simulink model "hw2Q7_model"  (R2021a)
settings: Solver=VariableStepAuto  StartTime=0.0  StopTime=time_end  RelTol=1e-3
values from neighbouring files (symbols this model uses):
  alpha = 60    [hw2Q7.m]
  E = 720    [hw2Q7.m]
  F = 180    [hw2Q7.m]
  K1 = (1 + G * K2) / G    [hw2Q7.m]
  K2 = K2_list{i}    [hw2Q7.m]
  m = 1000    [hw2Q7.m]
settings Model: Creator=kaiyu  LastModifiedBy=kaiyu

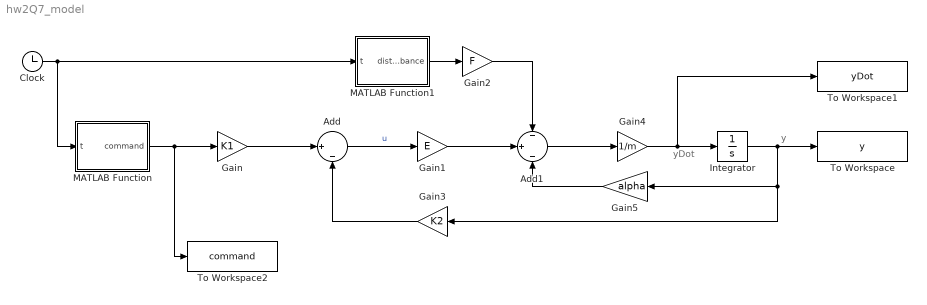
== system hw2Q7_model ==
  note: yDot
  note: y
  Add : Sum  Inputs=||+|-
  Add1 : Sum  Inputs=-|+|-
  Clock : Clock
  Gain : Gain  Gain=K1
  Gain1 : Gain  Gain=E
  Gain2 : Gain  Gain=F
  Gain3 : Gain  Gain=K2
  Gain4 : Gain  Gain=1/m
  Gain5 : Gain  Gain=alpha
  Integrator : Integrator  InitialCondition=20
  MATLAB Function : MATLAB Function  TreatAsAtomicUnit=on
  MATLAB Function1 : MATLAB Function  TreatAsAtomicUnit=on
  To Workspace : ToWorkspace  VariableName=y  SaveFormat=Timeseries  SampleTime=-1
  To Workspace1 : ToWorkspace  VariableName=yDot  SaveFormat=Timeseries  SampleTime=-1
  To Workspace2 : ToWorkspace  VariableName=command  SaveFormat=Timeseries  SampleTime=-1
  wires:
  Gain/1 -> Add/1
  Add/1 -> Gain1/1  "u"
  Gain1/1 -> Add1/2
  Gain2/1 -> Add1/1
  MATLAB Function1/1(disturbance) -> Gain2/1
  Clock/1 -> MATLAB Function/1(t), MATLAB Function1/1(t)
  Gain3/1 -> Add/2
  Add1/1 -> Gain4/1
  Integrator/1 -> Gain5/1, Gain3/1, To Workspace/1
  Gain5/1 -> Add1/3
  Gain4/1 -> To Workspace1/1, Integrator/1
  MATLAB Function/1(command) -> To Workspace2/1, Gain/1

== matlab function hw2Q7_model/MATLAB Function ==
  data: t input; command output
function command = r(t)
if (0 <= t) && (t < 5)
    out = 50;
elseif (5 <= t) && (t < 15)
    out = 55;
elseif (15 <= t) && (t < 25)
    out = 60;
elseif (25 <= t) && (t < 45)
    out = 60 - 4/3 * (t - 25);
else
    out = 45;
end

out = out * 1609.34 / 3600;     % Convert miles/hr to meters/sec
command = out;

== matlab function hw2Q7_model/MATLAB Function1 ==
  data: t input; disturbance output
function disturbance = d(t)
if (0 <= t) && (t < 35)
    out = 0;
elseif (35 <= t) && (t < 45)
    out = 1.3;
elseif (45 <= t) && (t < 55)
    out = 0;
elseif (55 <= t) && (t < 70)
    out = 5.0;
else
    out = 0;
end
disturbance = out;
